simulink model "bldc"  (R2023a)
settings: Solver=VariableStepAuto  StartTime=0.0  StopTime=30  RelTol=1e-3
libraries: spsMosfetLib x6, simulink x6, spsControlledVoltageSourceLib x1, spsGroundLib x1, slpidlib x1, spsPermanentMagnetSynchronousMachineLib x1, sps_lib x1
settings Model: Creator=Shrawani  LastModifiedBy=Shrawani

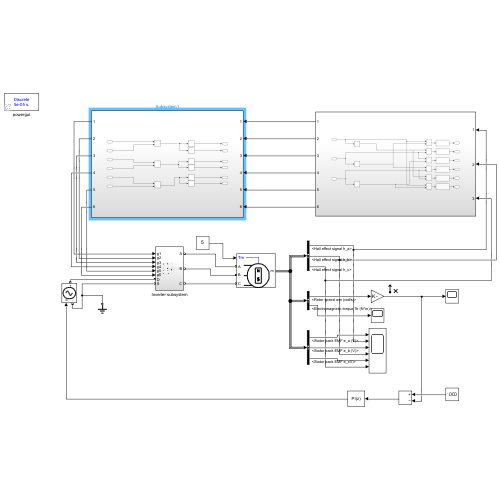
[thumbnail: Simulink's stored preview of the top-level diagram]
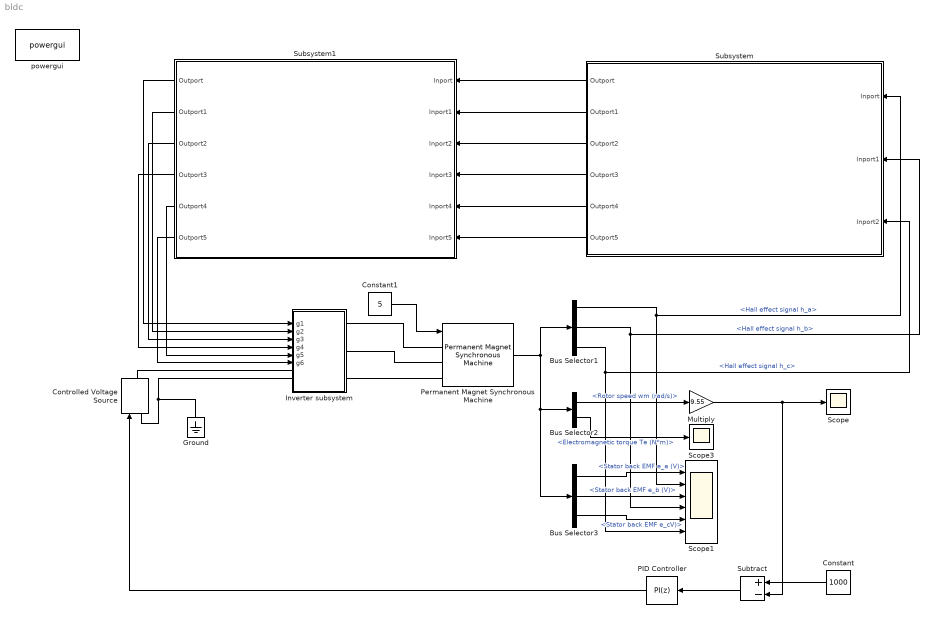
== system bldc ==
  Bus Selector1 : BusSelector  OutputSignals=Hall effect signal h_a,Hall effect signal h_b,Hall effect signal h_c
  Bus Selector2 : BusSelector  OutputSignals=Rotor speed wm (rad/s),Electromagnetic torque Te (N*m)
  Bus Selector3 : BusSelector  OutputSignals=Stator back EMF e_a (V),Stator back EMF e_b (V),Stator back EMF e_cV)
  Constant : Constant  Value=1000
  Constant1 : Constant  Value=5
  Controlled Voltage Source : spsControlledVoltageSourceLib/Controlled Voltage Source  Initialize=on  Source_Type=DC  Amplitude=200  Phase=0  Frequency=0  Measurements=None
  Ground : spsGroundLib/Ground  LConnTagsString=a
  Inverter subsystem : Subsystem
  Multiply : Gain  Gain=9.55
  PID Controller : slpidlib/PID Controller  Controller=PI  Form=Parallel  TimeDomain=Discrete-time  UseExternalTs=off  SampleTime=-1  IntegratorMethod=Forward Euler  FilterMethod=Forward Euler  ControllerParametersSource=internal  P=0.079782  I=5.286932  UseKiTs=off  D=500  N=0  UseFilter=on  TunerSelectOption=Transfer Function Based (PID Tuner App)  InitialConditionSource=internal  InitialConditionForIntegrator=0  InitialConditionForFilter=0  DifferentiatorICPrevScaledInput=0  ExternalReset=none  TrackingMode=off  Kt=1  LimitOutput=off  SatLimitsSource=internal  UpperSaturationLimit=inf  LowerSaturationLimit=-inf  LinearizeAsGain=on  AntiWindupMode=none  Kb=1  LimitIntegrator=off  UpperIntegratorSaturationLimit=inf  LowerIntegratorSaturationLimit=-inf  POutMin=[]  POutMax=[]  IOutMin=[]  IOutMax=[]  DOutMin=[]  DOutMax=[]  NOutMin=[]  NOutMax=[]  SumOutMin=[]  SumOutMax=[]  SaturationOutMin=[]  SaturationOutMax=[]  PParamMin=[]  PParamMax=[]  IParamMin=[]  IParamMax=[]  DParamMin=[]  DParamMax=[]  NParamMin=[]  NParamMax=[]  KbParamMin=[]  KbParamMax=[]  KtParamMin=[]  KtParamMax=[]  KbOutMin=[]  KbOutMax=[]  KtOutMin=[]  KtOutMax=[]  IntegratorOutMin=[]  IntegratorOutMax=[]  FilterOutMin=[]  FilterOutMax=[]  SumI1OutMin=[]  SumI1OutMax=[]  SumI2OutMin=[]  SumI2OutMax=[]  SumI3OutMin=[]  SumI3OutMax=[]  SumI4OutMin=[]  SumI4OutMax=[]  SumDOutMin=[]  SumDOutMax=[]  DifferentiatorOutMin=[]  DifferentiatorOutMax=[]  FilterDiffOutCoefMin=[]  FilterDiffOutCoefMax=[]  ReciprocalOutMin=[]  ReciprocalOutMax=[]  SumDenOutMin=[]  SumDenOutMax=[]  SumNumOutMin=[]  SumNumOutMax=[]  DivideOutMin=[]  DivideOutMax=[]  UdiffTsProdOutMin=[]  UdiffTsProdOutMax=[]  NTsProdOutMin=[]  NTsProdOutMax=[]  UintegralTsProdOutMin=[]  UintegralTsProdOutMax=[]  UngainTsProdOutMin=[]  UngainTsProdOutMax=[]  ClampingZeroOutDataTypeStr=Inherit: Inherit via back propagation  ClampingZeroOutMin=[]  ClampingZeroOutMax=[]  FilterDenConstantOutDataTypeStr=Inherit: Inherit via back propagation  FilterDenConstantOutMin=[]  FilterDenConstantOutMax=[]  PCopyOutDataTypeStr=Inherit: Inherit via back propagation  PCopyOutMin=[]  PCopyOutMax=[]  NCopyOutDataTypeStr=Inherit: Inherit via back propagation  NCopyOutMin=[]  NCopyOutMax=[]  IntegratorContinuousStateAttributes=''  IntegratorStateIdentifier=''  IntegratorStateMustResolveToSignalObject=off  IntegratorRTWStateStorageClass=Auto  FilterContinuousStateAttributes=''  FilterStateMustResolveToSignalObject=off  FilterRTWStateStorageClass=Auto  ParallelPVariant=InternalParameters  IdealPVariant=Disabled  IVariant=InternalParameters  DVariant=Disabled  IntegratorVariant=Discrete  SatVariant=Disabled  AWVariant=Passthrough  PCopyVariant=Disabled  TRVariant=Disabled  FdbkBlocksVariant=Forward  IdealPFdbkVariant=Disabled  SatFdbkVariant=Disabled  DerivativeFilterVariant=Disabled  NVariant=Disabled  NCopyVariant=Disabled_SignalSpec  FilterICVariant=Disabled  IntegratorICVariant=InternalICs  ExternalResetVariant=Disabled  TRSumVariant=Passthrough  SumFdbkVariant=Disabled  SumVariant=Sum_PI  TsampFilterVariant=InternalTs  TsampNgainVariant=Passthrough  TsampIntegralVariant=Disabled_SignalSpec  ExternalSaturationOutDataTypeStr=Inherit: Same as second input
  Permanent Magnet Synchronous Machine : spsPermanentMagnetSynchronousMachineLib/Permanent Magnet Synchronous Machine  NbPhases=3  FluxDistribution=Trapezoidal  RotorType=Round  MechanicalLoad=Torque Tm  PresetModel=No  ShowDetailedParameters=on  MeasurementBus=off  Resistance=1.43  Inductance=9.4e-3  dqInductances=[8.5e-3,8.5e-3]  La=0.000395  MachineConstant=Flux linkage established by magnets (V.s)  Flux=0.1194  VoltageCst=100.0283  TorqueCst=0.9552  Flat=120  Mechanical=[0.0027 0.0004924 4 0]  PolePairs=4  InitialConditions=[0,0, 0,0]  InitialConditions5ph=[0 0 0 0 0 0]  RefAngle=90 degrees behind phase A axis (modified Park)  IterativeDiscreteModel=Trapezoidal non iterative  TsBlock=-1  TsPowergui=0
  Scope : Scope
  Scope1 : Scope  NumInputPorts=6
  Scope3 : Scope
  Subsystem : Subsystem
  Subsystem1 : Subsystem
  Subtract : Sum  Inputs=+-
  powergui : sps_lib/powergui  Priority=1  SimulationMode=Discrete  SampleTime=50e-6  frequency=60  Iterations=50  frequencyindice=0  Pbase=100e6  ErrMax=1e-4  UnitsV=kV  UnitsW=MW  buscounter=0  FunctionMessages=off  echomessages=off  EnableUseOfTLC=off  CurrentSourceSwitches=off  DisableSnubberDevices=off  DisableRonSwitches=off  DisableVfSwitches=off  DisplayEquations=off  AutomaticDiscreteSolvers=off  SolverType=Tustin/Backward Euler (TBE)  Interpol=off  ExternalGateDelay=off  methode=off  Ts=100  x0status=blocks  SPID=on  SwTol=0  HookPort=off  NonlinearTolerance=1e-4  nMaxIteration=100  ContinueOnMaxIteration=off  RestoreLinks=warning  ResistiveCurrentMeasurement=off  Frange=[0:2:500]  Ylog=off  Xlog=on  ShowGrid=off  save=off  variable=ZData  structure=0  ZoomFFT=off  StartTime=0.0  cycles=1  DisplayStyle=1  fundamental=60  FreqAxis=off  MaxFrequency=1000  frequencyindicesteady=1  RmsSteady=1  display=off
  wires:
  Multiply/1 -> Subtract/2, Scope/1
  Subsystem1/4(Outport3) -> Inverter subsystem/4(g4)
  Bus Selector2/2 -> Scope3/1  "<Electromagnetic torque Te (N*m)>"
  Subsystem1/6(Outport5) -> Inverter subsystem/6(g6)
  Subsystem1/3(Outport2) -> Inverter subsystem/3(g3)
  Subsystem1/5(Outport4) -> Inverter subsystem/5(g5)
  Bus Selector3/1 -> Scope1/1  "<Stator back EMF e_a (V)>"
  Subsystem/1(Outport) -> Subsystem1/1(Inport)
  Subsystem/5(Outport4) -> Subsystem1/5(Inport4)
  Subsystem/3(Outport2) -> Subsystem1/3(Inport2)
  Bus Selector3/3 -> Scope1/5  "<Stator back EMF e_cV)>"
  Bus Selector2/1 -> Multiply/1  "<Rotor speed wm (rad/s)>"
  Constant1/1 -> Permanent Magnet Synchronous Machine/1
  Bus Selector3/2 -> Scope1/3  "<Stator back EMF e_b (V)>"
  Bus Selector1/3 -> Scope1/6, Subsystem/3(Inport2)  "<Hall effect signal h_c>"
  Subsystem1/2(Outport1) -> Inverter subsystem/2(g2)
  Subsystem1/1(Outport) -> Inverter subsystem/1(g1)
  Permanent Magnet Synchronous Machine/1 -> Bus Selector3/1, Bus Selector2/1, Bus Selector1/1
  Subsystem/4(Outport3) -> Subsystem1/4(Inport3)
  Subsystem/2(Outport1) -> Subsystem1/2(Inport1)
  Bus Selector1/2 -> Scope1/4, Subsystem/2(Inport1)  "<Hall effect signal h_b>"
  Subsystem/6(Outport5) -> Subsystem1/6(Inport5)
  Bus Selector1/1 -> Subsystem/1(Inport), Scope1/2  "<Hall effect signal h_a>"
  Constant/1 -> Subtract/1
  Subtract/1 -> PID Controller/1
  PID Controller/1 -> Controlled Voltage Source/1
  connections:
  Inverter subsystem/LConn2 -- Controlled Voltage Source/LConn1 -- Ground/LConn1
  Inverter subsystem/LConn1 -- Controlled Voltage Source/RConn1
  Inverter subsystem/RConn1 -- Permanent Magnet Synchronous Machine/LConn1
  Inverter subsystem/RConn2 -- Permanent Magnet Synchronous Machine/LConn2
  Inverter subsystem/RConn3 -- Permanent Magnet Synchronous Machine/LConn3

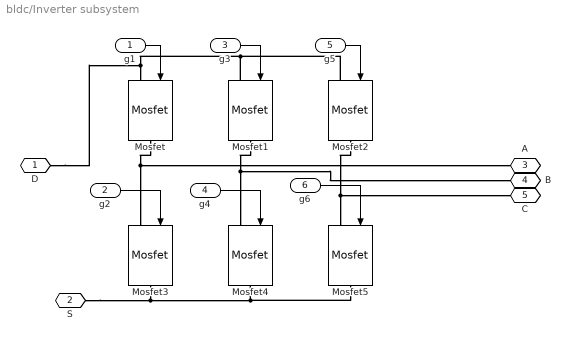
== system bldc/Inverter subsystem ==
  g1 : Inport
  g2 : Inport  Port=2
  g3 : Inport  Port=3
  g4 : Inport  Port=4
  g5 : Inport  Port=5
  g6 : Inport  Port=6
  Mosfet{,1..5} (6 alike) : spsMosfetLib/Mosfet  Ron=0.1  Lon=0  Rd=0.01  Vfd=0  IC=0  Rs=1e5  Cs=inf  Measurements=off
  D : PMIOPort  Side=Left
  S : PMIOPort  Port=2  Side=Left
  A : PMIOPort  Port=3  Side=Right
  B : PMIOPort  Port=4  Side=Right
  C : PMIOPort  Port=5  Side=Right
  wires:
  g2/1 -> Mosfet3/1
  g1/1 -> Mosfet/1
  g5/1 -> Mosfet2/1
  g6/1 -> Mosfet5/1
  g3/1 -> Mosfet1/1
  g4/1 -> Mosfet4/1
  connections:
  Mosfet/LConn1 -- Mosfet2/LConn1 -- Mosfet1/LConn1 -- D/RConn1
  Mosfet/RConn1 -- Mosfet3/LConn1 -- A/RConn1
  Mosfet1/RConn1 -- Mosfet4/LConn1 -- B/RConn1
  Mosfet2/RConn1 -- Mosfet5/LConn1 -- C/RConn1
  Mosfet3/RConn1 -- S/RConn1 -- Mosfet5/RConn1 -- Mosfet4/RConn1

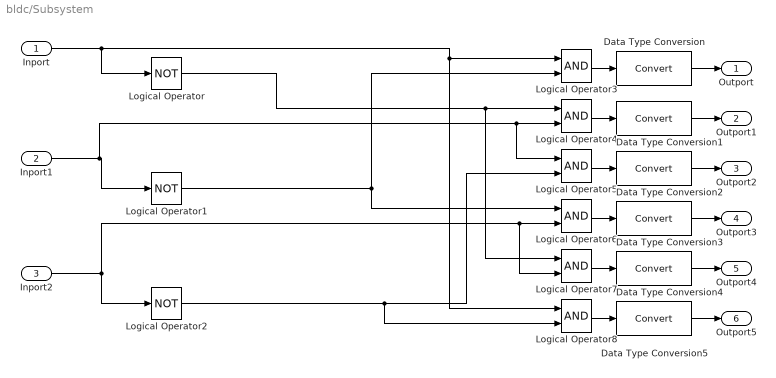
== system bldc/Subsystem ==
  Inport : Inport
  Inport1 : Inport  Port=2
  Inport2 : Inport  Port=3
  Data Type Conversion{,1..5} (6 alike) : DataTypeConversion  SaturateOnIntegerOverflow=off  RndMeth=Floor
  Logical Operator : Logic  Operator=NOT  AllPortsSameDT=off  OutDataTypeStr=boolean
  Logical Operator1 : Logic  Operator=NOT  AllPortsSameDT=off  OutDataTypeStr=boolean
  Logical Operator2 : Logic  Operator=NOT  AllPortsSameDT=off  OutDataTypeStr=boolean
  Logical Operator{3..8} (6 alike) : Logic  AllPortsSameDT=off  OutDataTypeStr=boolean
  Outport : Outport
  Outport1 : Outport  Port=2
  Outport2 : Outport  Port=3
  Outport3 : Outport  Port=4
  Outport4 : Outport  Port=5
  Outport5 : Outport  Port=6
  wires:
  Inport2/1 -> Logical Operator7/2, Logical Operator6/2, Logical Operator2/1
  Inport1/1 -> Logical Operator5/1, Logical Operator4/2, Logical Operator1/1
  Inport/1 -> Logical Operator8/1, Logical Operator3/1, Logical Operator/1
  Logical Operator1/1 -> Logical Operator3/2, Logical Operator6/1
  Logical Operator/1 -> Logical Operator7/1, Logical Operator4/1
  Logical Operator2/1 -> Logical Operator8/2, Logical Operator5/2
  Logical Operator3/1 -> Data Type Conversion/1
  Data Type Conversion/1 -> Outport/1
  Logical Operator4/1 -> Data Type Conversion1/1
  Data Type Conversion1/1 -> Outport1/1
  Logical Operator5/1 -> Data Type Conversion2/1
  Data Type Conversion2/1 -> Outport2/1
  Logical Operator6/1 -> Data Type Conversion3/1
  Data Type Conversion3/1 -> Outport3/1
  Logical Operator7/1 -> Data Type Conversion4/1
  Data Type Conversion4/1 -> Outport4/1
  Logical Operator8/1 -> Data Type Conversion5/1
  Data Type Conversion5/1 -> Outport5/1

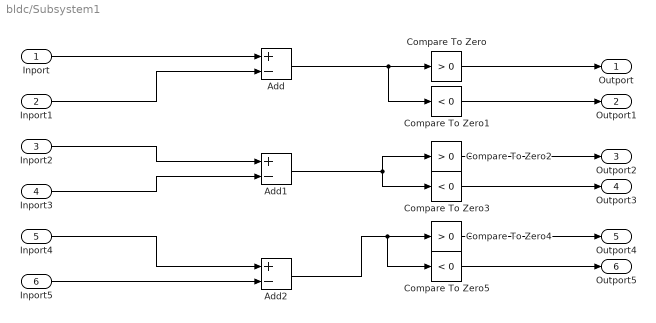
== system bldc/Subsystem1 ==
  Inport : Inport
  Inport1 : Inport  Port=2
  Inport2 : Inport  Port=3
  Inport3 : Inport  Port=4
  Inport4 : Inport  Port=5
  Inport5 : Inport  Port=6
  Add : Sum  Inputs=+-
  Add1 : Sum  Inputs=+-
  Add2 : Sum  Inputs=+-
  Compare To Zero : simulink/Logic and Bit Operations/Compare To Zero  relop=>  OutDataTypeStr=boolean
  Compare To Zero1 : simulink/Logic and Bit Operations/Compare To Zero  relop=<  OutDataTypeStr=boolean
  Compare To Zero2 : simulink/Logic and Bit Operations/Compare To Zero  relop=>  OutDataTypeStr=boolean
  Compare To Zero3 : simulink/Logic and Bit Operations/Compare To Zero  relop=<  OutDataTypeStr=boolean
  Compare To Zero4 : simulink/Logic and Bit Operations/Compare To Zero  relop=>  OutDataTypeStr=boolean
  Compare To Zero5 : simulink/Logic and Bit Operations/Compare To Zero  relop=<  OutDataTypeStr=boolean
  Outport : Outport
  Outport1 : Outport  Port=2
  Outport2 : Outport  Port=3
  Outport3 : Outport  Port=4
  Outport4 : Outport  Port=5
  Outport5 : Outport  Port=6
  wires:
  Add/1 -> Compare To Zero1/1, Compare To Zero/1
  Add1/1 -> Compare To Zero2/1, Compare To Zero3/1
  Add2/1 -> Compare To Zero5/1, Compare To Zero4/1
  Inport/1 -> Add/1
  Inport1/1 -> Add/2
  Inport2/1 -> Add1/1
  Inport3/1 -> Add1/2
  Inport4/1 -> Add2/1
  Inport5/1 -> Add2/2
  Compare To Zero/1 -> Outport/1
  Compare To Zero1/1 -> Outport1/1
  Compare To Zero2/1 -> Outport2/1
  Compare To Zero3/1 -> Outport3/1
  Compare To Zero4/1 -> Outport4/1
  Compare To Zero5/1 -> Outport5/1
